simulink model "EMS"  (R2024b)
settings: Solver=FixedStepAuto  StartTime=0.0  StopTime=10.0  RelTol=1e-3  EnableMultiTasking=on
undefined symbols (not defined in the file): EAccumulatorCapacity, NEnduranceLaps
libraries: simulink x26
settings Model: DataDictionary=Master_Dictionary.sldd  EnableAccessToBaseWorkspace=off  Creator=torni  LastModifiedBy=Will
settings OptimizationCC: DefaultParameterBehavior=Inlined  EnhancedBackFolding=on  PassReuseOutputArgsAs=Individual arguments  ZeroExternalMemoryAtStartup=off  ZeroInternalMemoryAtStartup=off  MaxStackSize=8192  OptimizeBlockOrder=speed  DifferentSizesBufferReuse=on  OptimizationCustomize=off  EfficientTunableParamExpr=on
settings DebuggingCC: ParameterTunabilityLossMsg=error
settings HardwareCC: ProdBitPerPointer=32  ProdBitPerSizeT=32  ProdBitPerPtrDiffT=32  ProdLargestAtomicInteger=Long  ProdLargestAtomicFloat=Double  ProdWordSize=32  ProdLongLongMode=on  ProdHWDeviceType=ARM Compatible->ARM Cortex-M
settings SFSimCC: MATLABDynamicMemAlloc=off
settings RTWCC: Description=Embedded Coder  SystemTargetFile=ert.tlc  HardwareBoard=STM32H7xx Based (Single-core)  TemplateMakefile=ert_default_tmf  Toolchain=GNU Tools for ARM Embedded Processors
settings CodeAppCC: ForceParamTrailComments=on  IgnoreCustomStorageClasses=off  OperatorAnnotations=on  SimulinkDataObjDesc=on  SFDataObjDesc=on  InsertBlockDesc=on
settings ERTTargetCC: TargetLangStandard=C99 (ISO)  CodeReplacementLibrary=ARM Cortex-M  ExtModeTransport=3  ExtModeStaticAlloc=on  ExtModeStaticAllocSize=2048  ExtModeMexFile=ext_xcp  ExtModeIntrfLevel=Level2 - Open

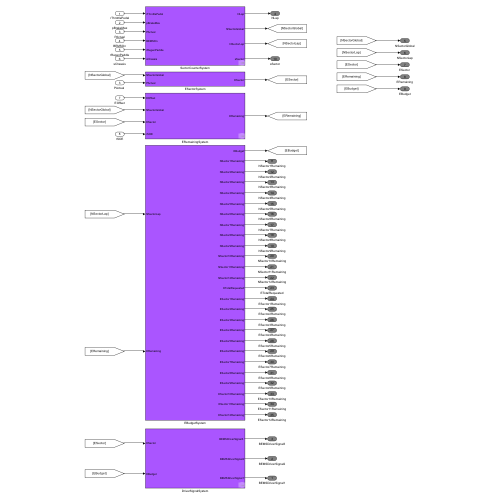
[thumbnail: Simulink's stored preview of the top-level diagram]
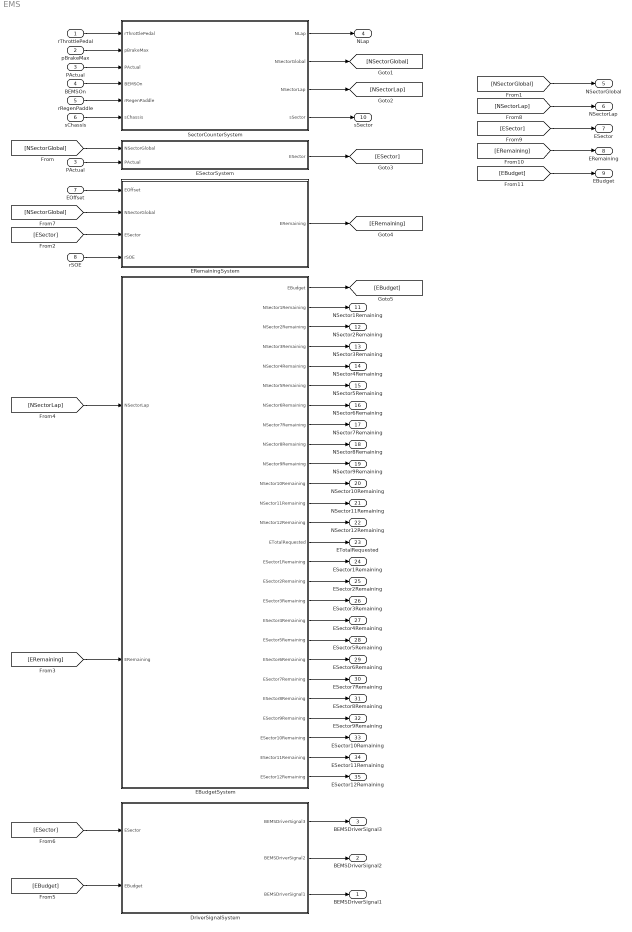
== system EMS ==
  rThrottlePedal : Inport
  pBrakeMax : Inport  Port=2
  PActual : Inport  Port=3
  BEMSOn : Inport  Port=4
  rRegenPaddle : Inport  Port=5
  sChassis : Inport  Port=6
  EOffset : Inport  Port=7
  rSOE : Inport  Port=8
  DriverSignalSystem : Subsystem
  EBudgetSystem : Subsystem
  ERemainingSystem : Subsystem
  ESectorSystem : Subsystem
  "PActual " : InportShadow  Port=3
  SectorCounterSystem : Subsystem
  BEMSDriverSignal1 : Outport  VectorParamsAs1DForOutWhenUnconnected=off
  BEMSDriverSignal2 : Outport  Port=2  VectorParamsAs1DForOutWhenUnconnected=off
  BEMSDriverSignal3 : Outport  Port=3  VectorParamsAs1DForOutWhenUnconnected=off
  NLap : Outport  Port=4  VectorParamsAs1DForOutWhenUnconnected=off
  NSectorGlobal : Outport  Port=5  VectorParamsAs1DForOutWhenUnconnected=off
  NSectorLap : Outport  Port=6  VectorParamsAs1DForOutWhenUnconnected=off
  "ESector " : Outport  Port=7  VectorParamsAs1DForOutWhenUnconnected=off
  ERemaining : Outport  Port=8  VectorParamsAs1DForOutWhenUnconnected=off
  EBudget : Outport  Port=9  VectorParamsAs1DForOutWhenUnconnected=off
  sSector : Outport  Port=10  VectorParamsAs1DForOutWhenUnconnected=off
  NSector1Remaining : Outport  Port=11  VectorParamsAs1DForOutWhenUnconnected=off
  NSector2Remaining : Outport  Port=12  VectorParamsAs1DForOutWhenUnconnected=off
  NSector3Remaining : Outport  Port=13  VectorParamsAs1DForOutWhenUnconnected=off
  NSector4Remaining : Outport  Port=14  VectorParamsAs1DForOutWhenUnconnected=off
  NSector5Remaining : Outport  Port=15  VectorParamsAs1DForOutWhenUnconnected=off
  NSector6Remaining : Outport  Port=16  VectorParamsAs1DForOutWhenUnconnected=off
  NSector7Remaining : Outport  Port=17  VectorParamsAs1DForOutWhenUnconnected=off
  NSector8Remaining : Outport  Port=18  VectorParamsAs1DForOutWhenUnconnected=off
  NSector9Remaining : Outport  Port=19  VectorParamsAs1DForOutWhenUnconnected=off
  NSector10Remaining : Outport  Port=20  VectorParamsAs1DForOutWhenUnconnected=off
  NSector11Remaining : Outport  Port=21  VectorParamsAs1DForOutWhenUnconnected=off
  NSector12Remaining : Outport  Port=22  VectorParamsAs1DForOutWhenUnconnected=off
  ETotalRequested : Outport  Port=23  VectorParamsAs1DForOutWhenUnconnected=off
  ESector1Remaining : Outport  Port=24  VectorParamsAs1DForOutWhenUnconnected=off
  ESector2Remaining : Outport  Port=25  VectorParamsAs1DForOutWhenUnconnected=off
  ESector3Remaining : Outport  Port=26  VectorParamsAs1DForOutWhenUnconnected=off
  ESector4Remaining : Outport  Port=27  VectorParamsAs1DForOutWhenUnconnected=off
  ESector5Remaining : Outport  Port=28  VectorParamsAs1DForOutWhenUnconnected=off
  ESector6Remaining : Outport  Port=29  VectorParamsAs1DForOutWhenUnconnected=off
  ESector7Remaining : Outport  Port=30  VectorParamsAs1DForOutWhenUnconnected=off
  ESector8Remaining : Outport  Port=31  VectorParamsAs1DForOutWhenUnconnected=off
  ESector9Remaining : Outport  Port=32  VectorParamsAs1DForOutWhenUnconnected=off
  ESector10Remaining : Outport  Port=33  VectorParamsAs1DForOutWhenUnconnected=off
  ESector11Remaining : Outport  Port=34  VectorParamsAs1DForOutWhenUnconnected=off
  ESector12Remaining : Outport  Port=35  VectorParamsAs1DForOutWhenUnconnected=off
  wires:
  [NSectorGlobal] -> ESectorSystem/1(NSectorGlobal)
  DriverSignalSystem/3(BEMSDriverSignal1) -> BEMSDriverSignal1/1
  [ESector] -> "ESector "/1
  [EBudget] -> EBudget/1
  DriverSignalSystem/1("BEMSDriverSignal3 ") -> BEMSDriverSignal3/1
  SectorCounterSystem/3(NSectorLap) -> [NSectorLap]
  pBrakeMax/1 -> SectorCounterSystem/2(pBrakeMax)
  [EBudget] -> DriverSignalSystem/2(EBudget)
  rSOE/1 -> ERemainingSystem/4(rSOE)
  [ESector] -> DriverSignalSystem/1(ESector)
  [NSectorGlobal] -> NSectorGlobal/1
  SectorCounterSystem/4(sSector) -> sSector/1
  [NSectorLap] -> NSectorLap/1
  "PActual "/1 -> ESectorSystem/2(PActual)
  [ESector] -> ERemainingSystem/3(ESector)
  [NSectorGlobal] -> ERemainingSystem/2(NSectorGlobal)
  [NSectorLap] -> EBudgetSystem/1(NSectorLap)
  [ERemaining] -> EBudgetSystem/2(ERemaining)
  rRegenPaddle/1 -> SectorCounterSystem/5(rRegenPaddle)
  EOffset/1 -> ERemainingSystem/1(EOffset)
  EBudgetSystem/1(EBudget) -> [EBudget]
  ESectorSystem/1(ESector) -> [ESector]
  SectorCounterSystem/1(NLap) -> NLap/1
  DriverSignalSystem/2(BEMSDriverSignal2) -> BEMSDriverSignal2/1
  sChassis/1 -> SectorCounterSystem/6(sChassis)
  [ERemaining] -> ERemaining/1
  ERemainingSystem/1(ERemaining) -> [ERemaining]
  PActual/1 -> SectorCounterSystem/3(PActual)
  SectorCounterSystem/2(NSectorGlobal) -> [NSectorGlobal]
  BEMSOn/1 -> SectorCounterSystem/4(BEMSOn)
  EBudgetSystem/11(NSector10Remaining) -> NSector10Remaining/1
  EBudgetSystem/24(ESector10Remaining) -> ESector10Remaining/1
  EBudgetSystem/26(ESector12Remaining) -> ESector12Remaining/1
  EBudgetSystem/17(ESector3Remaining) -> ESector3Remaining/1
  EBudgetSystem/25(ESector11Remaining) -> ESector11Remaining/1
  EBudgetSystem/16(ESector2Remaining) -> ESector2Remaining/1
  EBudgetSystem/4(NSector3Remaining) -> NSector3Remaining/1
  EBudgetSystem/12(NSector11Remaining) -> NSector11Remaining/1
  EBudgetSystem/6(NSector5Remaining) -> NSector5Remaining/1
  EBudgetSystem/2(NSector1Remaining) -> NSector1Remaining/1
  EBudgetSystem/5(NSector4Remaining) -> NSector4Remaining/1
  EBudgetSystem/7(NSector6Remaining) -> NSector6Remaining/1
  EBudgetSystem/22(ESector8Remaining) -> ESector8Remaining/1
  EBudgetSystem/15(ESector1Remaining) -> ESector1Remaining/1
  EBudgetSystem/8(NSector7Remaining) -> NSector7Remaining/1
  EBudgetSystem/20(ESector6Remaining) -> ESector6Remaining/1
  EBudgetSystem/9(NSector8Remaining) -> NSector8Remaining/1
  EBudgetSystem/21(ESector7Remaining) -> ESector7Remaining/1
  EBudgetSystem/13(NSector12Remaining) -> NSector12Remaining/1
  EBudgetSystem/3(NSector2Remaining) -> NSector2Remaining/1
  EBudgetSystem/10(NSector9Remaining) -> NSector9Remaining/1
  EBudgetSystem/14(ETotalRequested) -> ETotalRequested/1
  EBudgetSystem/23(ESector9Remaining) -> ESector9Remaining/1
  EBudgetSystem/18(ESector4Remaining) -> ESector4Remaining/1
  EBudgetSystem/19(ESector5Remaining) -> ESector5Remaining/1
  rThrottlePedal/1 -> SectorCounterSystem/1(rThrottlePedal)

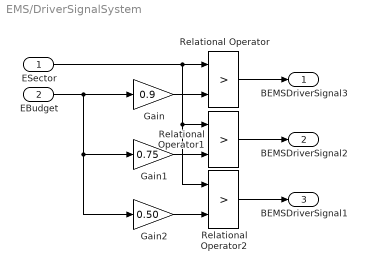
== system EMS/DriverSignalSystem ==
  ESector : Inport
  EBudget : Inport  Port=2
  Gain : Gain  Gain=0.9
  Gain1 : Gain  Gain=0.75
  Gain2 : Gain  Gain=0.50
  Relational Operator : RelationalOperator  Operator=>  OutDataTypeStr=boolean  RndMeth=Simplest  InputSameDT=off
  Relational Operator1 : RelationalOperator  Operator=>  OutDataTypeStr=boolean  RndMeth=Simplest  InputSameDT=off
  Relational Operator2 : RelationalOperator  Operator=>  OutDataTypeStr=boolean  RndMeth=Simplest  InputSameDT=off
  "BEMSDriverSignal3 " : Outport  VectorParamsAs1DForOutWhenUnconnected=off
  BEMSDriverSignal2 : Outport  Port=2  VectorParamsAs1DForOutWhenUnconnected=off
  BEMSDriverSignal1 : Outport  Port=3  VectorParamsAs1DForOutWhenUnconnected=off
  wires:
  EBudget/1 -> Gain2/1, Gain1/1, Gain/1
  Gain/1 -> Relational Operator/2
  ESector/1 -> Relational Operator/1, Relational Operator1/1, Relational Operator2/1
  Gain1/1 -> Relational Operator1/2
  Gain2/1 -> Relational Operator2/2
  Relational Operator/1 -> "BEMSDriverSignal3 "/1
  Relational Operator1/1 -> BEMSDriverSignal2/1
  Relational Operator2/1 -> BEMSDriverSignal1/1

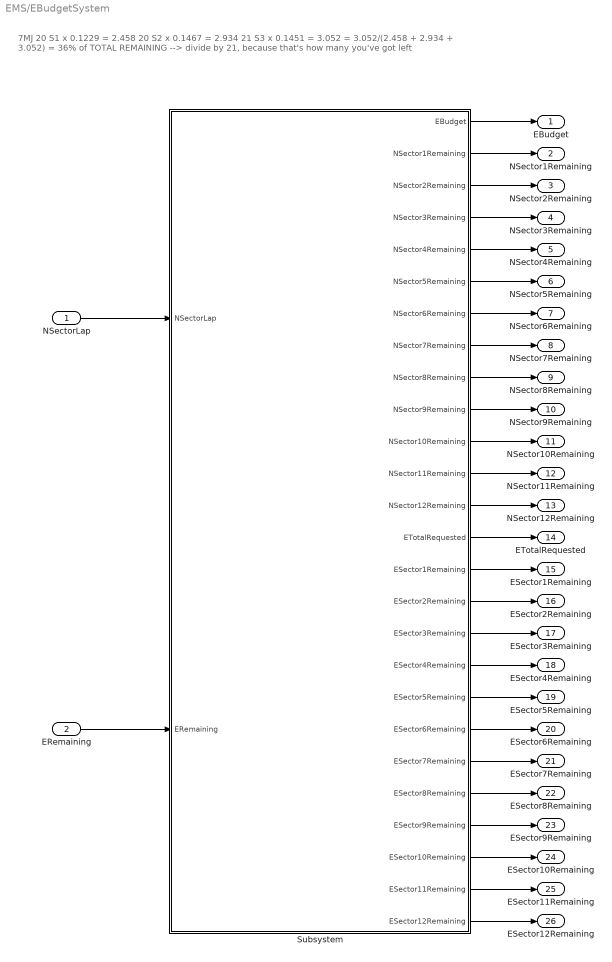
== system EMS/EBudgetSystem ==
  note: 7MJ
      | 20 S1 x 0.1229 = 2.458
      | 20 S2 x 0.1467 = 2.934
      | 21 S3 x 0.1451 = 3.052 = 3.052/(2.458 + 2.934 + 3.052) = 36% of TOTAL REMAINING --> divide by 21, because that's how many you've got left
  NSectorLap : Inport
  ERemaining : Inport  Port=2
  Subsystem : Subsystem
  EBudget : Outport  VectorParamsAs1DForOutWhenUnconnected=off
  NSector1Remaining : Outport  Port=2  VectorParamsAs1DForOutWhenUnconnected=off
  NSector2Remaining : Outport  Port=3  VectorParamsAs1DForOutWhenUnconnected=off
  NSector3Remaining : Outport  Port=4  VectorParamsAs1DForOutWhenUnconnected=off
  NSector4Remaining : Outport  Port=5  VectorParamsAs1DForOutWhenUnconnected=off
  NSector5Remaining : Outport  Port=6  VectorParamsAs1DForOutWhenUnconnected=off
  NSector6Remaining : Outport  Port=7  VectorParamsAs1DForOutWhenUnconnected=off
  NSector7Remaining : Outport  Port=8  VectorParamsAs1DForOutWhenUnconnected=off
  NSector8Remaining : Outport  Port=9  VectorParamsAs1DForOutWhenUnconnected=off
  NSector9Remaining : Outport  Port=10  VectorParamsAs1DForOutWhenUnconnected=off
  NSector10Remaining : Outport  Port=11  VectorParamsAs1DForOutWhenUnconnected=off
  NSector11Remaining : Outport  Port=12  VectorParamsAs1DForOutWhenUnconnected=off
  NSector12Remaining : Outport  Port=13  VectorParamsAs1DForOutWhenUnconnected=off
  ETotalRequested : Outport  Port=14  VectorParamsAs1DForOutWhenUnconnected=off
  ESector1Remaining : Outport  Port=15  VectorParamsAs1DForOutWhenUnconnected=off
  ESector2Remaining : Outport  Port=16  VectorParamsAs1DForOutWhenUnconnected=off
  ESector3Remaining : Outport  Port=17  VectorParamsAs1DForOutWhenUnconnected=off
  ESector4Remaining : Outport  Port=18  VectorParamsAs1DForOutWhenUnconnected=off
  ESector5Remaining : Outport  Port=19  VectorParamsAs1DForOutWhenUnconnected=off
  ESector6Remaining : Outport  Port=20  VectorParamsAs1DForOutWhenUnconnected=off
  ESector7Remaining : Outport  Port=21  VectorParamsAs1DForOutWhenUnconnected=off
  ESector8Remaining : Outport  Port=22  VectorParamsAs1DForOutWhenUnconnected=off
  ESector9Remaining : Outport  Port=23  VectorParamsAs1DForOutWhenUnconnected=off
  ESector10Remaining : Outport  Port=24  VectorParamsAs1DForOutWhenUnconnected=off
  ESector11Remaining : Outport  Port=25  VectorParamsAs1DForOutWhenUnconnected=off
  ESector12Remaining : Outport  Port=26  VectorParamsAs1DForOutWhenUnconnected=off
  wires:
  NSectorLap/1 -> Subsystem/1(NSectorLap)
  ERemaining/1 -> Subsystem/2(ERemaining)
  Subsystem/1(EBudget) -> EBudget/1
  Subsystem/3(NSector2Remaining) -> NSector2Remaining/1
  Subsystem/17(ESector3Remaining) -> ESector3Remaining/1
  Subsystem/18(ESector4Remaining) -> ESector4Remaining/1
  Subsystem/19(ESector5Remaining) -> ESector5Remaining/1
  Subsystem/20(ESector6Remaining) -> ESector6Remaining/1
  Subsystem/21(ESector7Remaining) -> ESector7Remaining/1
  Subsystem/22(ESector8Remaining) -> ESector8Remaining/1
  Subsystem/23(ESector9Remaining) -> ESector9Remaining/1
  Subsystem/24(ESector10Remaining) -> ESector10Remaining/1
  Subsystem/25(ESector11Remaining) -> ESector11Remaining/1
  Subsystem/26(ESector12Remaining) -> ESector12Remaining/1
  Subsystem/16(ESector2Remaining) -> ESector2Remaining/1
  Subsystem/15(ESector1Remaining) -> ESector1Remaining/1
  Subsystem/14(ETotalRequested) -> ETotalRequested/1
  Subsystem/13(NSector12Remaining) -> NSector12Remaining/1
  Subsystem/12(NSector11Remaining) -> NSector11Remaining/1
  Subsystem/11(NSector10Remaining) -> NSector10Remaining/1
  Subsystem/10(NSector9Remaining) -> NSector9Remaining/1
  Subsystem/8(NSector7Remaining) -> NSector7Remaining/1
  Subsystem/7(NSector6Remaining) -> NSector6Remaining/1
  Subsystem/6(NSector5Remaining) -> NSector5Remaining/1
  Subsystem/5(NSector4Remaining) -> NSector4Remaining/1
  Subsystem/4(NSector3Remaining) -> NSector3Remaining/1
  Subsystem/2(NSector1Remaining) -> NSector1Remaining/1
  Subsystem/9(NSector8Remaining) -> NSector8Remaining/1

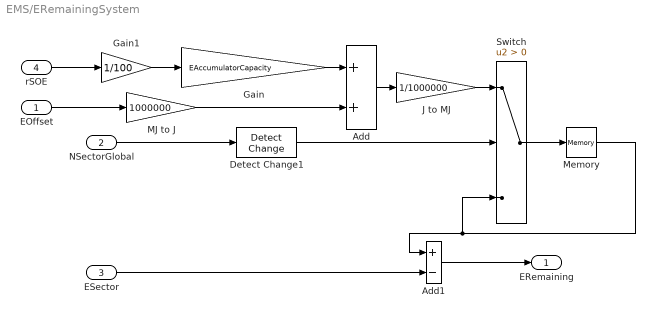
== system EMS/ERemainingSystem ==
  EOffset : Inport
  NSectorGlobal : Inport  Port=2
  ESector : Inport  Port=3  OutDataTypeStr=double
  rSOE : Inport  Port=4
  Add : Sum
  Add1 : Sum  Inputs=+-
  Detect Change1 : simulink/Logic and Bit Operations/Detect Change  vinit=1  OutDataTypeStr=boolean
  Gain : Gain  Gain=EAccumulatorCapacity
  Gain1 : Gain  Gain=1/100
  J to MJ : Gain  Gain=1/1000000
  MJ to J : Gain  Gain=1000000
  Memory : Memory  InheritSampleTime=on
  Switch : Switch  Criteria=u2 > Threshold  SaturateOnIntegerOverflow=off  InputSameDT=off
  ERemaining : Outport  VectorParamsAs1DForOutWhenUnconnected=off
  wires:
  NSectorGlobal/1 -> Detect Change1/1
  Switch/1 -> Memory/1
  Add/1 -> J to MJ/1
  ESector/1 -> Add1/2
  rSOE/1 -> Gain1/1
  Gain/1 -> Add/1
  Gain1/1 -> Gain/1
  Detect Change1/1 -> Switch/2
  Add1/1 -> ERemaining/1
  Memory/1 -> Switch/3, Add1/1
  EOffset/1 -> MJ to J/1
  MJ to J/1 -> Add/2
  J to MJ/1 -> Switch/1

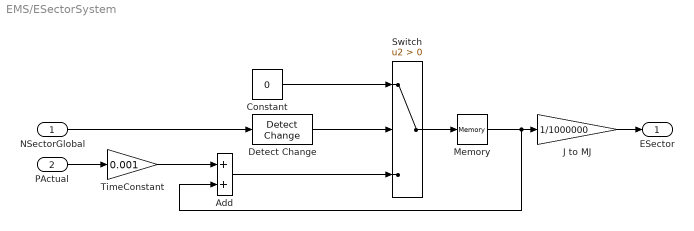
== system EMS/ESectorSystem ==
  NSectorGlobal : Inport
  PActual : Inport  Port=2
  Add : Sum
  Constant : Constant  Value=0
  Detect Change : simulink/Logic and Bit Operations/Detect Change  vinit=0  OutDataTypeStr=boolean
  J to MJ : Gain  Gain=1/1000000
  Memory : Memory  InheritSampleTime=on
  Switch : Switch  Criteria=u2 > Threshold  SaturateOnIntegerOverflow=off  InputSameDT=off
  TimeConstant : Gain  Gain=0.001
  ESector : Outport  VectorParamsAs1DForOutWhenUnconnected=off
  wires:
  Memory/1 -> J to MJ/1, Add/2
  TimeConstant/1 -> Add/1
  Detect Change/1 -> Switch/2
  Switch/1 -> Memory/1
  PActual/1 -> TimeConstant/1
  Add/1 -> Switch/3
  Constant/1 -> Switch/1
  NSectorGlobal/1 -> Detect Change/1
  J to MJ/1 -> ESector/1

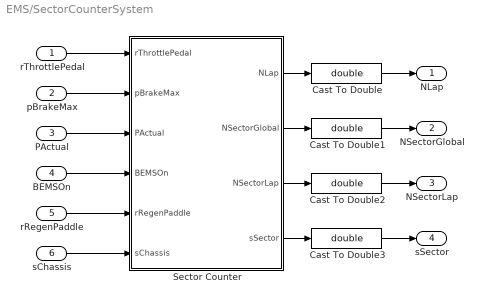
== system EMS/SectorCounterSystem ==
  rThrottlePedal : Inport  OutDataTypeStr=double
  pBrakeMax : Inport  Port=2  OutDataTypeStr=double
  PActual : Inport  Port=3  OutDataTypeStr=double
  BEMSOn : Inport  Port=4  OutDataTypeStr=boolean
  rRegenPaddle : Inport  Port=5  OutDataTypeStr=double
  sChassis : Inport  Port=6  OutDataTypeStr=double
  Cast To Double{,1..3} (4 alike) : DataTypeConversion  OutDataTypeStr=double  SaturateOnIntegerOverflow=off  RndMeth=Floor
  Sector Counter : Stateflow chart  TreatAsAtomicUnit=on
  NLap : Outport  VectorParamsAs1DForOutWhenUnconnected=off
  NSectorGlobal : Outport  Port=2  VectorParamsAs1DForOutWhenUnconnected=off
  NSectorLap : Outport  Port=3  VectorParamsAs1DForOutWhenUnconnected=off
  sSector : Outport  Port=4  VectorParamsAs1DForOutWhenUnconnected=off
  wires:
  Sector Counter/4(sSector) -> Cast To Double3/1
  Cast To Double2/1 -> NSectorLap/1
  Cast To Double/1 -> NLap/1
  Sector Counter/2(NSectorGlobal) -> Cast To Double1/1
  Cast To Double1/1 -> NSectorGlobal/1
  Sector Counter/1(NLap) -> Cast To Double/1
  Sector Counter/3(NSectorLap) -> Cast To Double2/1
  Cast To Double3/1 -> sSector/1
  rThrottlePedal/1 -> Sector Counter/1(rThrottlePedal)
  pBrakeMax/1 -> Sector Counter/2(pBrakeMax)
  PActual/1 -> Sector Counter/3(PActual)
  rRegenPaddle/1 -> Sector Counter/5(rRegenPaddle)
  sChassis/1 -> Sector Counter/6(sChassis)
  BEMSOn/1 -> Sector Counter/4(BEMSOn)

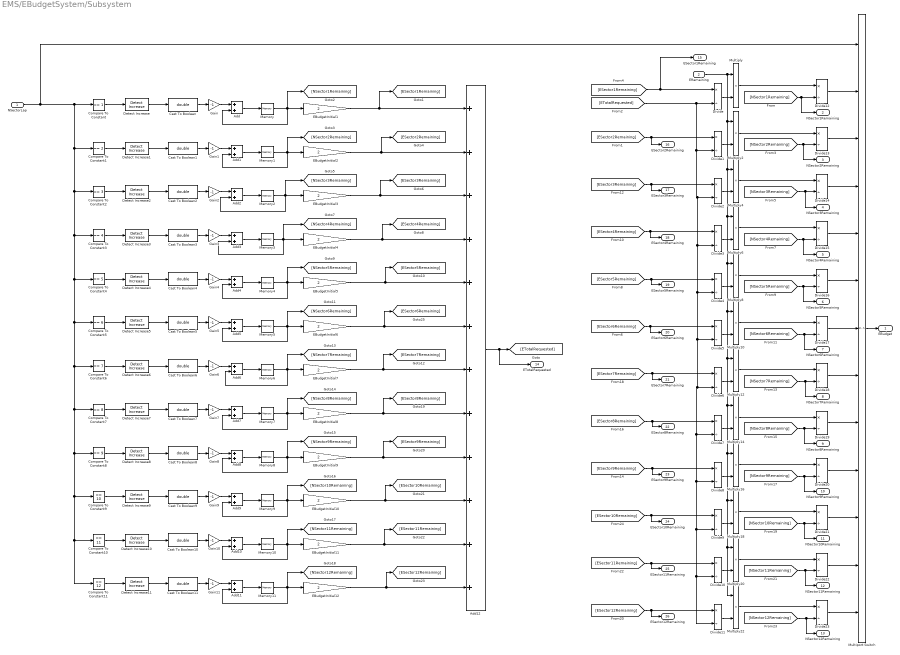
== system EMS/EBudgetSystem/Subsystem ==
  NSectorLap : Inport
  ERemaining : Inport  Port=2
  Add{,1..11} (12 alike) : Sum
  Add12 : Sum  Inputs=12
  Cast To Boolean{,1..11} (12 alike) : DataTypeConversion  OutDataTypeStr=double  SaturateOnIntegerOverflow=off  RndMeth=Floor
  Compare To Constant : simulink/Logic and Bit Operations/Compare To Constant  relop===  const=1  OutDataTypeStr=boolean
  Compare To Constant1 : simulink/Logic and Bit Operations/Compare To Constant  relop===  const=2  OutDataTypeStr=boolean
  Compare To Constant10 : simulink/Logic and Bit Operations/Compare To Constant  relop===  const=11  OutDataTypeStr=boolean
  Compare To Constant11 : simulink/Logic and Bit Operations/Compare To Constant  relop===  const=12  OutDataTypeStr=boolean
  Compare To Constant2 : simulink/Logic and Bit Operations/Compare To Constant  relop===  const=3  OutDataTypeStr=boolean
  Compare To Constant3 : simulink/Logic and Bit Operations/Compare To Constant  relop===  const=4  OutDataTypeStr=boolean
  Compare To Constant4 : simulink/Logic and Bit Operations/Compare To Constant  relop===  const=5  OutDataTypeStr=boolean
  Compare To Constant5 : simulink/Logic and Bit Operations/Compare To Constant  relop===  const=6  OutDataTypeStr=boolean
  Compare To Constant6 : simulink/Logic and Bit Operations/Compare To Constant  relop===  const=7  OutDataTypeStr=boolean
  Compare To Constant7 : simulink/Logic and Bit Operations/Compare To Constant  relop===  const=8  OutDataTypeStr=boolean
  Compare To Constant8 : simulink/Logic and Bit Operations/Compare To Constant  relop===  const=9  OutDataTypeStr=boolean
  Compare To Constant9 : simulink/Logic and Bit Operations/Compare To Constant  relop===  const=10  OutDataTypeStr=boolean
  Detect Increase{,1..11} (12 alike) : simulink/Logic and Bit Operations/Detect Increase  vinit=0  OutDataTypeStr=boolean
  Divide{,1..23} (24 alike) : Product  Inputs=*/
  EBudgetInitial{1..12} (12 alike) : Gain  Gain=2  OutDataTypeStr=double
  Gain{,1..11} (12 alike) : Gain  Gain=-1
  Memory{,1..11} (12 alike) : Memory  InitialCondition=NEnduranceLaps  InheritSampleTime=on
  Multiply{,2,4,6,8,10,12,14,16,18,20,22} (12 alike) : Product
  Multiport Switch : MultiPortSwitch  Inputs=12  SaturateOnIntegerOverflow=off  InputSameDT=off
  EBudget : Outport  VectorParamsAs1DForOutWhenUnconnected=off
  NSector1Remaining : Outport  Port=2  VectorParamsAs1DForOutWhenUnconnected=off
  NSector2Remaining : Outport  Port=3  VectorParamsAs1DForOutWhenUnconnected=off
  NSector3Remaining : Outport  Port=4  VectorParamsAs1DForOutWhenUnconnected=off
  NSector4Remaining : Outport  Port=5  VectorParamsAs1DForOutWhenUnconnected=off
  NSector5Remaining : Outport  Port=6  VectorParamsAs1DForOutWhenUnconnected=off
  NSector6Remaining : Outport  Port=7  VectorParamsAs1DForOutWhenUnconnected=off
  NSector7Remaining : Outport  Port=8  VectorParamsAs1DForOutWhenUnconnected=off
  NSector8Remaining : Outport  Port=9  VectorParamsAs1DForOutWhenUnconnected=off
  NSector9Remaining : Outport  Port=10  VectorParamsAs1DForOutWhenUnconnected=off
  NSector10Remaining : Outport  Port=11  VectorParamsAs1DForOutWhenUnconnected=off
  NSector11Remaining : Outport  Port=12  VectorParamsAs1DForOutWhenUnconnected=off
  NSector12Remaining : Outport  Port=13  VectorParamsAs1DForOutWhenUnconnected=off
  ETotalRequested : Outport  Port=14  VectorParamsAs1DForOutWhenUnconnected=off
  ESector1Remaining : Outport  Port=15  VectorParamsAs1DForOutWhenUnconnected=off
  ESector2Remaining : Outport  Port=16  VectorParamsAs1DForOutWhenUnconnected=off
  ESector3Remaining : Outport  Port=17  VectorParamsAs1DForOutWhenUnconnected=off
  ESector4Remaining : Outport  Port=18  VectorParamsAs1DForOutWhenUnconnected=off
  ESector5Remaining : Outport  Port=19  VectorParamsAs1DForOutWhenUnconnected=off
  ESector6Remaining : Outport  Port=20  VectorParamsAs1DForOutWhenUnconnected=off
  ESector7Remaining : Outport  Port=21  VectorParamsAs1DForOutWhenUnconnected=off
  ESector8Remaining : Outport  Port=22  VectorParamsAs1DForOutWhenUnconnected=off
  ESector9Remaining : Outport  Port=23  VectorParamsAs1DForOutWhenUnconnected=off
  ESector10Remaining : Outport  Port=24  VectorParamsAs1DForOutWhenUnconnected=off
  ESector11Remaining : Outport  Port=25  VectorParamsAs1DForOutWhenUnconnected=off
  ESector12Remaining : Outport  Port=26  VectorParamsAs1DForOutWhenUnconnected=off
  wires:
  Memory/1 -> [NSector1Remaining], EBudgetInitial1/1, Add/2
  Detect Increase/1 -> Cast To Boolean/1
  Add/1 -> Memory/1
  Compare To Constant/1 -> Detect Increase/1
  Gain/1 -> Add/1
  Memory1/1 -> EBudgetInitial2/1, Add1/2, [NSector2Remaining]
  Detect Increase1/1 -> Cast To Boolean1/1
  Add1/1 -> Memory1/1
  Compare To Constant1/1 -> Detect Increase1/1
  Gain1/1 -> Add1/1
  Memory2/1 -> EBudgetInitial3/1, [NSector3Remaining], Add2/2
  Detect Increase2/1 -> Cast To Boolean2/1
  Add2/1 -> Memory2/1
  Compare To Constant2/1 -> Detect Increase2/1
  Gain2/1 -> Add2/1
  Memory3/1 -> EBudgetInitial4/1, [NSector4Remaining], Add3/2
  Detect Increase3/1 -> Cast To Boolean3/1
  Add3/1 -> Memory3/1
  Compare To Constant3/1 -> Detect Increase3/1
  Gain3/1 -> Add3/1
  Memory4/1 -> EBudgetInitial5/1, [NSector5Remaining], Add4/2
  Detect Increase4/1 -> Cast To Boolean4/1
  Add4/1 -> Memory4/1
  Compare To Constant4/1 -> Detect Increase4/1
  Gain4/1 -> Add4/1
  Memory5/1 -> EBudgetInitial6/1, [NSector6Remaining], Add5/2
  Detect Increase5/1 -> Cast To Boolean5/1
  Add5/1 -> Memory5/1
  Compare To Constant5/1 -> Detect Increase5/1
  Gain5/1 -> Add5/1
  Memory6/1 -> EBudgetInitial7/1, [NSector7Remaining], Add6/2
  Detect Increase6/1 -> Cast To Boolean6/1
  Add6/1 -> Memory6/1
  Compare To Constant6/1 -> Detect Increase6/1
  Gain6/1 -> Add6/1
  Memory7/1 -> EBudgetInitial8/1, [NSector8Remaining], Add7/2
  Detect Increase7/1 -> Cast To Boolean7/1
  Add7/1 -> Memory7/1
  Compare To Constant7/1 -> Detect Increase7/1
  Gain7/1 -> Add7/1
  Memory8/1 -> EBudgetInitial9/1, [NSector9Remaining], Add8/2
  Detect Increase8/1 -> Cast To Boolean8/1
  Add8/1 -> Memory8/1
  Compare To Constant8/1 -> Detect Increase8/1
  Gain8/1 -> Add8/1
  Memory9/1 -> EBudgetInitial10/1, [NSector10Remaining], Add9/2
  Detect Increase9/1 -> Cast To Boolean9/1
  Add9/1 -> Memory9/1
  Compare To Constant9/1 -> Detect Increase9/1
  Gain9/1 -> Add9/1
  Memory10/1 -> EBudgetInitial11/1, [NSector11Remaining], Add10/2
  Detect Increase10/1 -> Cast To Boolean10/1
  Add10/1 -> Memory10/1
  Compare To Constant10/1 -> Detect Increase10/1
  Gain10/1 -> Add10/1
  Memory11/1 -> EBudgetInitial12/1, [NSector12Remaining], Add11/2
  Detect Increase11/1 -> Cast To Boolean11/1
  Add11/1 -> Memory11/1
  Compare To Constant11/1 -> Detect Increase11/1
  NSectorLap/1 -> Compare To Constant6/1, Compare To Constant7/1, Compare To Constant8/1, Compare To Constant9/1, Compare To Constant11/1, Compare To Constant10/1, Compare To Constant5/1, Compare To Constant4/1, Compare To Constant3/1, Compare To Constant2/1, Compare To Constant1/1, Compare To Constant/1, Multiport Switch/1
  Gain11/1 -> Add11/1
  EBudgetInitial12/1 -> [ESector12Remaining], Add12/12
  EBudgetInitial11/1 -> [ESector11Remaining], Add12/11
  EBudgetInitial10/1 -> [ESector10Remaining], Add12/10
  EBudgetInitial9/1 -> [ESector9Remaining], Add12/9
  EBudgetInitial8/1 -> [ESector8Remaining], Add12/8
  EBudgetInitial7/1 -> [ESector7Remaining], Add12/7
  EBudgetInitial5/1 -> [ESector5Remaining], Add12/5
  EBudgetInitial4/1 -> [ESector4Remaining], Add12/4
  EBudgetInitial3/1 -> [ESector3Remaining], Add12/3
  EBudgetInitial2/1 -> [ESector2Remaining], Add12/2
  EBudgetInitial1/1 -> [ESector1Remaining], Add12/1
  Add12/1 -> ETotalRequested/1, [ETotalRequested]
  EBudgetInitial6/1 -> [ESector6Remaining], Add12/6
  [NSector1Remaining] -> NSector1Remaining/1, Divide12/2
  [ESector1Remaining] -> ESector1Remaining/1, Divide/1
  Multiply/1 -> Divide12/1
  Divide/1 -> Multiply/2
  Divide12/1 -> Multiport Switch/2
  ERemaining/1 -> Multiply22/1, Multiply20/1, Multiply18/1, Multiply16/1, Multiply14/1, Multiply12/1, Multiply10/1, Multiply8/1, Multiply6/1, Multiply4/1, Multiply2/1, Multiply/1
  Divide1/1 -> Multiply2/2
  Multiply2/1 -> Divide13/1
  [ESector2Remaining] -> ESector2Remaining/1, Divide1/1
  [NSector2Remaining] -> NSector2Remaining/1, Divide13/2
  Divide13/1 -> Multiport Switch/3
  [NSector3Remaining] -> NSector3Remaining/1, Divide14/2
  Divide2/1 -> Multiply4/2
  Multiply4/1 -> Divide14/1
  [ESector3Remaining] -> ESector3Remaining/1, Divide2/1
  Divide14/1 -> Multiport Switch/4
  [NSector4Remaining] -> NSector4Remaining/1, Divide15/2
  Divide3/1 -> Multiply6/2
  Multiply6/1 -> Divide15/1
  [ESector4Remaining] -> ESector4Remaining/1, Divide3/1
  Divide15/1 -> Multiport Switch/5
  [NSector5Remaining] -> NSector5Remaining/1, Divide16/2
  Divide4/1 -> Multiply8/2
  Multiply8/1 -> Divide16/1
  [ESector5Remaining] -> ESector5Remaining/1, Divide4/1
  Divide16/1 -> Multiport Switch/6
  [NSector6Remaining] -> NSector6Remaining/1, Divide17/2
  Divide5/1 -> Multiply10/2
  Multiply10/1 -> Divide17/1
  [ESector6Remaining] -> ESector6Remaining/1, Divide5/1
  Divide17/1 -> Multiport Switch/7
  [ESector7Remaining] -> ESector7Remaining/1, Divide6/1
  Divide6/1 -> Multiply12/2
  Multiply12/1 -> Divide18/1
  [NSector7Remaining] -> NSector7Remaining/1, Divide18/2
  Divide18/1 -> Multiport Switch/8
  [ESector8Remaining] -> ESector8Remaining/1, Divide7/1
  Divide7/1 -> Multiply14/2
  Multiply14/1 -> Divide19/1
  [NSector8Remaining] -> NSector8Remaining/1, Divide19/2
  Divide19/1 -> Multiport Switch/9
  [ESector9Remaining] -> ESector9Remaining/1, Divide8/1
  Divide8/1 -> Multiply16/2
  Multiply16/1 -> Divide20/1
  [NSector9Remaining] -> NSector9Remaining/1, Divide20/2
  Divide20/1 -> Multiport Switch/10
  [ESector10Remaining] -> ESector10Remaining/1, Divide9/1
  Divide9/1 -> Multiply18/2
  Multiply18/1 -> Divide21/1
  [NSector10Remaining] -> NSector10Remaining/1, Divide21/2
  Divide21/1 -> Multiport Switch/11
  [ESector11Remaining] -> ESector11Remaining/1, Divide10/1
  Divide10/1 -> Multiply20/2
  Multiply20/1 -> Divide22/1
  [NSector11Remaining] -> NSector11Remaining/1, Divide22/2
  Divide22/1 -> Multiport Switch/12
  [ESector12Remaining] -> ESector12Remaining/1, Divide11/1
  [ETotalRequested] -> Divide11/2, Divide10/2, Divide9/2, Divide8/2, Divide7/2, Divide6/2, Divide5/2, Divide4/2, Divide3/2, Divide2/2, Divide1/2, Divide/2
  Divide11/1 -> Multiply22/2
  Multiply22/1 -> Divide23/1
  [NSector12Remaining] -> NSector12Remaining/1, Divide23/2
  Divide23/1 -> Multiport Switch/13
  Cast To Boolean/1 -> Gain/1
  Cast To Boolean1/1 -> Gain1/1
  Cast To Boolean2/1 -> Gain2/1
  Cast To Boolean3/1 -> Gain3/1
  Cast To Boolean4/1 -> Gain4/1
  Cast To Boolean5/1 -> Gain5/1
  Cast To Boolean6/1 -> Gain6/1
  Cast To Boolean7/1 -> Gain7/1
  Cast To Boolean8/1 -> Gain8/1
  Cast To Boolean9/1 -> Gain9/1
  Cast To Boolean10/1 -> Gain10/1
  Cast To Boolean11/1 -> Gain11/1
  Multiport Switch/1 -> EBudget/1

== stateflow chart EMS/SectorCounterSystem/Sector Counter ==
  state Start
    entry:
    NLap=0;
    NSectorLap=1;
    NSectorGlobal=0;
  state Wait_
    NSectorLap==1;
    NSectorGlobal=1;
    sSector=0;
  state Sector1
    entry:
    NSectorLap=1;
    NSectorGlobal=NSectorGlobal+1;
  state Wait_12
    entry:
    sSector=sChassis;
    NLap=NLap+1;
  state Sector3
    entry:
    NSectorLap=NSectorLap+1;
    NSectorGlobal=NSectorGlobal+1;
  state Sector2
    entry:
    NSectorLap=NSectorLap+1;
    NSectorGlobal=NSectorGlobal+1;
  state Wait_1
    entry:
    sSector=sChassis;
  state Wait_2
    entry:
    sSector=sChassis;
  state Wait_3
    entry:
    sSector=sChassis;
  state Sector4
    entry:
    NSectorLap=NSectorLap+1;
    NSectorGlobal=NSectorGlobal+1;
  state Sector12
    entry:
    NSectorLap=NSectorLap+1;
    NSectorGlobal=NSectorGlobal+1;
  state Wait_4
    entry:
    sSector=sChassis;
  state Wait_11
    entry:
    sSector=sChassis;
  state Sector5
    entry:
    NSectorLap=NSectorLap+1;
    NSectorGlobal=NSectorGlobal+1;
  state Sector11
    entry:
    NSectorLap=NSectorLap+1;
    NSectorGlobal=NSectorGlobal+1;
  state Wait_5
    entry:
    sSector=sChassis;
  state Wait_10
    entry:
    sSector=sChassis;
  state Sector6
    entry:
    NSectorLap=NSectorLap+1;
    NSectorGlobal=NSectorGlobal+1;
  state Sector10
    entry:
    NSectorLap=NSectorLap+1;
    NSectorGlobal=NSectorGlobal+1;
  state Sector9
    entry:
    NSectorLap=NSectorLap+1;
    NSectorGlobal=NSectorGlobal+1;
  state Sector8
    entry:
    NSectorLap=NSectorLap+1;
    NSectorGlobal=NSectorGlobal+1;
  state Sector7
    entry:
    NSectorLap=NSectorLap+1;
    NSectorGlobal=NSectorGlobal+1;
  state Wait_9
    entry:
    sSector=sChassis;
  state Wait_8
    entry:
    sSector=sChassis;
  state Wait_7
    entry:
    sSector=sChassis;
  state Wait_6
    entry:
    sSector=sChassis;
  (default) -> Start
  Start -> Wait_ : [BEMSOn==1]
  Wait_ -> Sector1 : [rThrottlePedal>10&&PActual>2]
  Wait_12 -> Sector1 : [rThrottlePedal>10&&PActual>2]
  Sector1 -> Wait_1 : [(rRegenPaddle>10||pBrakeMax>3)&&(sChassis-sSector>=77)]
  Sector12 -> Wait_12 : [(rRegenPaddle>10||pBrakeMax>3)&&(sChassis-sSector>=36)]
  Wait_2 -> Sector3 : [rThrottlePedal>10&&PActual>2]
  Sector3 -> Wait_3 : [(rRegenPaddle>10||pBrakeMax>3)&&(sChassis-sSector>=101)]
  Sector2 -> Wait_2 : [(rRegenPaddle>10||pBrakeMax>3)&&(sChassis-sSector>=71)]
  Wait_1 -> Sector2 : [rThrottlePedal>10&&PActual>2]
  Wait_3 -> Sector4 : [rThrottlePedal>10&&PActual>2]
  Sector4 -> Wait_4 : [(rRegenPaddle>10||pBrakeMax>3)&&(sChassis-sSector>=40)]
  Wait_11 -> Sector12 : [rThrottlePedal>10&&PActual>2]
  Wait_4 -> Sector5 : [rThrottlePedal>10&&PActual>2]
  Sector11 -> Wait_11 : [(rRegenPaddle>10||pBrakeMax>3)&&(sChassis-sSector>=29)]
  Sector5 -> Wait_5 : [(rRegenPaddle>10||pBrakeMax>3)&&(sChassis-sSector>=35)]
  Wait_10 -> Sector11 : [rThrottlePedal>10&&PActual>2]
  Wait_5 -> Sector6 : [rThrottlePedal>10&&PActual>2]
  Sector10 -> Wait_10 : [(rRegenPaddle>10||pBrakeMax>3)&&(sChassis-sSector>=40)]
  Sector6 -> Wait_6 : [(rRegenPaddle>10||pBrakeMax>3)&&(sChassis-sSector>=41)]
  Wait_9 -> Sector10 : [rThrottlePedal>10&&PActual>2]
  Sector8 -> Wait_8 : [(rRegenPaddle>10||pBrakeMax>3)&&(sChassis-sSector>=49)]
  Sector7 -> Wait_7 : [(rRegenPaddle>10||pBrakeMax>3)&&(sChassis-sSector>=64)]
  Sector9 -> Wait_9 : [(rRegenPaddle>10||pBrakeMax>3)&&(sChassis-sSector>=106)]
  Wait_7 -> Sector8 : [rThrottlePedal>10&&PActual>2]
  Wait_6 -> Sector7 : [rThrottlePedal>10&&PActual>2]
  Wait_8 -> Sector9 : [rThrottlePedal>10&&PActual>2]
  data: NLap output double =0; rThrottlePedal input double; pBrakeMax input double; PActual input double; BEMSOn input; NSectorGlobal output double =0; NSectorLap output double =0; rRegenPaddle input double; sChassis input double; sSector output
